simulink model "adaptive_mpc_simulink"  (R2019a)
settings: Solver=VariableStepAuto  StartTime=0.0  StopTime=30  RelTol=1e-3
libraries: mpclib x1
settings Model: Creator=alexh  LastModifiedBy=alexh

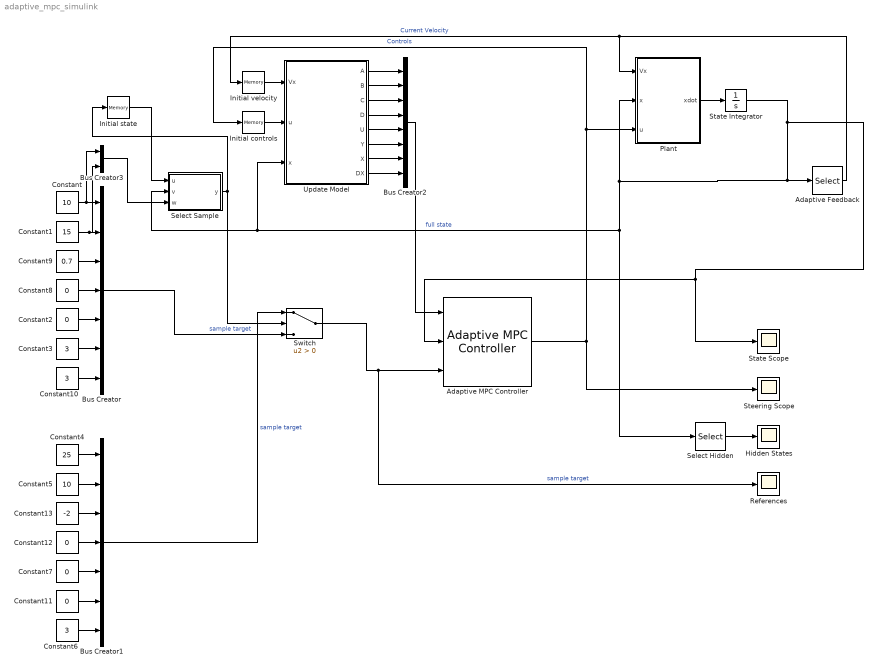
== system adaptive_mpc_simulink ==
  Adaptive Feedback : Selector  InputPortWidth=7  IndexOptions=Index vector (dialog)  Indices=[6]  OutputSizes=1
  Adaptive MPC Controller : mpclib/Adaptive MPC Controller  SCDEnableBlockLinearizationSpecification=on  mpcobj=blind_mpc  enable_value=0  updateMPCinCallerWorkspace=on  md_inport=off  mv_inport=off  uref_inport=off  return_cost=off  return_mvseq=off  return_qpstatus=off  return_xseq=off  return_state=off  return_ovseq=off  state_inport=off  isltv_plant=off  umin_inport=off  umax_inport=off  ymin_inport=off  ymax_inport=off  cc_inport=off  ywt_inport=off  uwt_inport=off  duwt_inport=off  rhoeps_inport=off  pm_inport=off  MaximumP=10  HorizonChoice=FixedHorizon  BlockDataType=double  SampleTimeInherited=off  switch_inport=off
      settings: SourceProductName=MATLAB Runtime - Model Predictive Control Toolbox Addin  SourceProductBaseCode=Missing
  Bus Creator3 : BusCreator  Inputs=2
  Bus Creator : BusCreator  Inputs=7
  Bus Creator1 : BusCreator  Inputs=7
  Bus Creator2 : BusCreator  Inputs=8
  Constant : Constant  Value=10
  Constant1 : Constant  Value=15
  Constant10 : Constant  Value=3
  Constant{2,7..8,11..12} (5 alike) : Constant  Value=0
  Constant13 : Constant  Value=-2
  Constant3 : Constant  Value=3
  Constant4 : Constant  Value=25
  Constant5 : Constant  Value=10
  Constant6 : Constant  Value=3
  Constant9 : Constant  Value=0.7
  Hidden States : Scope
  Initial controls : Memory
  Initial state : Memory
  Initial velocity : Memory  InitialCondition=1
  Plant : MATLAB Function  TreatAsAtomicUnit=on
  References : Scope
  Select Hidden : Selector  InputPortWidth=7  IndexOptions=Index vector (dialog)  Indices=[4 5]  OutputSizes=1
  Select Sample : MATLAB Function  TreatAsAtomicUnit=on
  State Integrator : Integrator  ContinuousStateAttributes='vehicleState'
  State Scope : Scope
  Steering Scope : Scope
  Switch : Switch  Criteria=u2 > Threshold
  Update Model : MATLAB Function  TreatAsAtomicUnit=on
  wires:
  Adaptive MPC Controller/1 -> Initial controls/1, Plant/3(u), Steering Scope/1  "Controls"
  Plant/1(xdot) -> State Integrator/1
  State Integrator/1 -> Adaptive MPC Controller/2, State Scope/1, Plant/2(x), Select Hidden/1, Select Sample/2(v), Update Model/3(x), Adaptive Feedback/1  "full state"
  Constant1/1 -> Bus Creator3/2, Bus Creator/2
  Switch/1 -> Adaptive MPC Controller/3, References/1  "sample target"
  Update Model/8(DX) -> Bus Creator2/8
  Update Model/1(A) -> Bus Creator2/1
  Update Model/2(B) -> Bus Creator2/2
  Update Model/3(C) -> Bus Creator2/3
  Update Model/4(D) -> Bus Creator2/4
  Update Model/5(U) -> Bus Creator2/5
  Update Model/6(Y) -> Bus Creator2/6
  Update Model/7(X) -> Bus Creator2/7
  Bus Creator2/1 -> Adaptive MPC Controller/1
  Initial controls/1 -> Update Model/2(u)
  Adaptive Feedback/1 -> Plant/1(Vx), Initial velocity/1  "Current Velocity"
  Initial velocity/1 -> Update Model/1(Vx)
  Select Hidden/1 -> Hidden States/1
  Select Sample/1(y) -> Initial state/1, Switch/2
  Constant/1 -> Bus Creator3/1, Bus Creator/1
  Bus Creator3/1 -> Select Sample/3(w)
  Initial state/1 -> Select Sample/1(u)
  Constant9/1 -> Bus Creator/3
  Constant3/1 -> Bus Creator/6
  Constant8/1 -> Bus Creator/4
  Constant2/1 -> Bus Creator/5
  Constant10/1 -> Bus Creator/7
  Constant12/1 -> Bus Creator1/4
  Constant11/1 -> Bus Creator1/6
  Bus Creator1/1 -> Switch/1  "sample target"
  Constant4/1 -> Bus Creator1/1
  Constant13/1 -> Bus Creator1/3
  Constant6/1 -> Bus Creator1/7
  Constant5/1 -> Bus Creator1/2
  Constant7/1 -> Bus Creator1/5
  Bus Creator/1 -> Switch/3  "sample target"

== matlab function adaptive_mpc_simulink/Update Model ==
  data: Vx input; u input; A output; x input; B output; C output; D output; U output; Y output; X output; DX output
function [A,B,C,D,U,Y,X,DX] = fcn(Vx,u,x)

if( Vx < 0.01)
    Vx = 0.01;
end

m = 30;     % Mass
lf = 0.7;   % Distance mass center/front wheel
lr = 0.3;   % Distance mass center/rear wheel
cf = 300;   % Cornering Stiffness front
cr = 300;   % Cornering Stiffness rear
iz = 100;   % Yaw Moment of Innertia?
Ts = 0.1;

factor_y = sin(x(3)+ x(5));
factor_x = cos(x(3)+ x(5));

Ac = [0, 0, -Vx, 0, -1, 1, 0;   %  Very crude spaceholder calc for x pos
    %v0, 0, 0, 0, 0, factor_x;
    0, 0, Vx, 0, 1, 0, 0;
    % 0, 0, 0, 0, 0, factor_y;
    0, 0, 0, 1, 0, 0, 0;
    0, 0, 0, -1/Vx*(cf*lf^2+cr*lr^2)/iz, -(cf*lf-cr*lr)/iz, 0, 0;
    0, 0, 0, -1-1/Vx^2*(cf*lf-cr*lr)/m, -1/Vx*(cf+cr)/m, 0, 0;
    0, 0, 0, 0, 0, -.1, 0;        % Very crude definition of speed
    0, 0, 0, 0, 0, -1, 0
    ];

Bc = [0, 0, 0, 2*cf*lf/iz, 2*cf/m, 0, 0;    % Steering angle
    0, 0, 0, 0, 0, 1, 0;
    0, 0, 0, 0, 0, -2, 0]';                 % acceleration/break

Cc = [1, 0, 0, 0, 0, 0, 0;
    0, 1, 0, 0, 0, 0, 0;
    0, 0, 1, 0, 0, 0, 0;
    0, 0, 0, 1, 0, 0, 0;
    0, 0, 0, 0, 1, 0, 0;
    0, 0, 0, 0, 0, 1, 0;
    0, 0, 0, 0, 0, 0, 1];


Dc = zeros(7,3);

% Generate discrete-time model
nx = size(Ac,1);
nu = size(Bc,2);
M = expm([[Ac Bc]*Ts; zeros(nu,nx+nu)]);
A = M(1:nx,1:nx);
B = M(1:nx,nx+1:nx+nu);
C = Cc;
D = Dc;

% Nominal conditions for discrete-time plant
X = x';
U = u';
Y = (C*x + D*u)';
DX = (A*x+B*u-x)';
%DX = [0, 0, 0, 0, 0, 0];

% Should be 6x1
% A 6x6 x=6x1
% B 6x2 u=2x1

== matlab function adaptive_mpc_simulink/Plant ==
  data: Vx input; x input; u input; xdot output
function xdot = fcn(Vx, x, u)

if (Vx < 0.01) 
    Vx = 0.01;
end

factor_y = sin(x(3)+ x(5));
factor_x = cos(x(3)+ x(5));

m = 30;     % Mass
lf = 0.7;   % Distance mass center/front wheel
lr = 0.3;   % Distance mass center/rear wheel
cf = 300;   % Cornering Stiffness front
cr = 300;   % Cornering Stiffness rear
iz = 100;   % Yaw Moment of Innertia?
Ts = 0.1;

% Continuous-time model
A = [0, 0, -Vx, 0, -1, 1, 0;   %  Very crude spaceholder calc for x pos
    % 0, 0, 0, 0, 0, factor_x;
    0, 0, Vx, 0, 1, 0, 0;
    % 0, 0, 0, 0, 0, factor_y;
    0, 0, 0, 1, 0, 0, 0;
    0, 0, 0, -1/Vx*(cf*lf^2+cr*lr^2)/iz, -(cf*lf-cr*lr)/iz, 0, 0;
    0, 0, 0, -1-1/Vx^2*(cf*lf-cr*lr)/m, -1/Vx*(cf+cr)/m, 0, 0;
    0, 0, 0, 0, 0, -.1, 0;      % Very crude definition of speed
    0, 0, 0, 0, 0, -1, 0
    ];

B = [0, 0, 0, 2*cf*lf/iz, 2*cf/m, 0, 0;    % Steering angle
    0, 0, 0, 0, 0, 1, 0;
    0, 0, 0, 0, 0, -2, 0]';                 % acceleration/break

xdot = A*x + B*u;

== matlab function adaptive_mpc_simulink/Select Sample ==
  data: u input; y output; v input; w input
function y = fcn(u, v, w)

if u==1
    y = 1;
elseif (w(1)-v(1) < 1) && (w(2)-v(2) < 1)
    y = 1;
else
    y = 0;
end
